simulink model "transerFunction1_PP"  (R2015a)
settings: Solver=ode45  StartTime=0.0  StopTime=10.0  RelTol=1e-3
settings Model: Creator=teme  LastModifiedBy=Teme

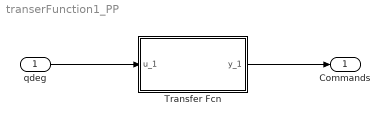
== system transerFunction1_PP ==
  qdeg : Inport  RequirementInfo={} %GIDa_6b9ebac5_2580_4efd_a5b0_351cee0e55a8  OutDataTypeStr=double
  Transfer Fcn : Subsystem  TreatAsAtomicUnit=on
  Commands : Outport  RequirementInfo={} %GIDa_15f1b71d_d2b6_4fce_a512_ded7c92776f4
  wires:
  qdeg/1 -> Transfer Fcn/1(u_1)
  Transfer Fcn/1(y_1) -> Commands/1

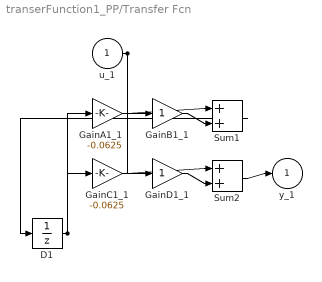
== system transerFunction1_PP/Transfer Fcn ==
  u_1 : Inport  OutDataTypeStr=double
  D1 : UnitDelay  SampleTime=0.01
  GainA1_1 : Gain  Gain=-0.0625  SaturateOnIntegerOverflow=on  OutDataTypeStr=Inherit: Same as input  ParamDataTypeStr=Inherit: Same as input
  GainB1_1 : Gain  SaturateOnIntegerOverflow=on  OutDataTypeStr=Inherit: Same as input  ParamDataTypeStr=Inherit: Same as input
  GainC1_1 : Gain  Gain=-0.0625  SaturateOnIntegerOverflow=on  OutDataTypeStr=Inherit: Same as input  ParamDataTypeStr=Inherit: Same as input
  GainD1_1 : Gain  SaturateOnIntegerOverflow=on  OutDataTypeStr=Inherit: Same as input  ParamDataTypeStr=Inherit: Same as input
  Sum1 : Sum  SaturateOnIntegerOverflow=on  InputSameDT=on  OutDataTypeStr=Inherit: Same as first input
  Sum2 : Sum  SaturateOnIntegerOverflow=on  InputSameDT=on  OutDataTypeStr=Inherit: Same as first input
  y_1 : Outport
  wires:
  Sum2/1 -> y_1/1
  Sum1/1 -> D1/1
  GainD1_1/1 -> Sum2/2
  GainB1_1/1 -> Sum1/2
  u_1/1 -> GainD1_1/1, GainB1_1/1
  GainC1_1/1 -> Sum2/1
  GainA1_1/1 -> Sum1/1
  D1/1 -> GainC1_1/1, GainA1_1/1
